simulink model "NEM_DVPP_OPEN"  (R2024a)
settings: Solver=ode23tb  StartTime=0.0  StopTime=60  RelTol=1e-3
libraries: simulink x1
settings Model: Creator=aidan  LastModifiedBy=aidan

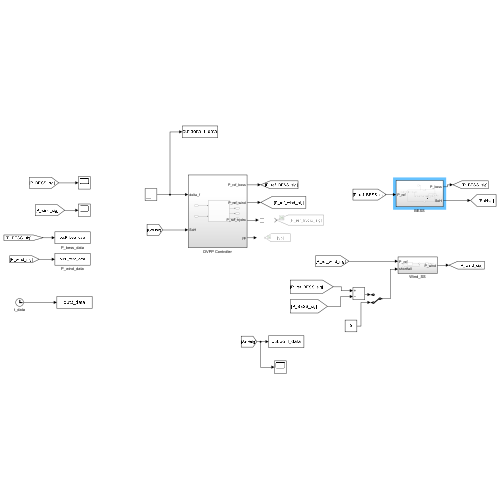
[thumbnail: Simulink's stored preview of the top-level diagram]
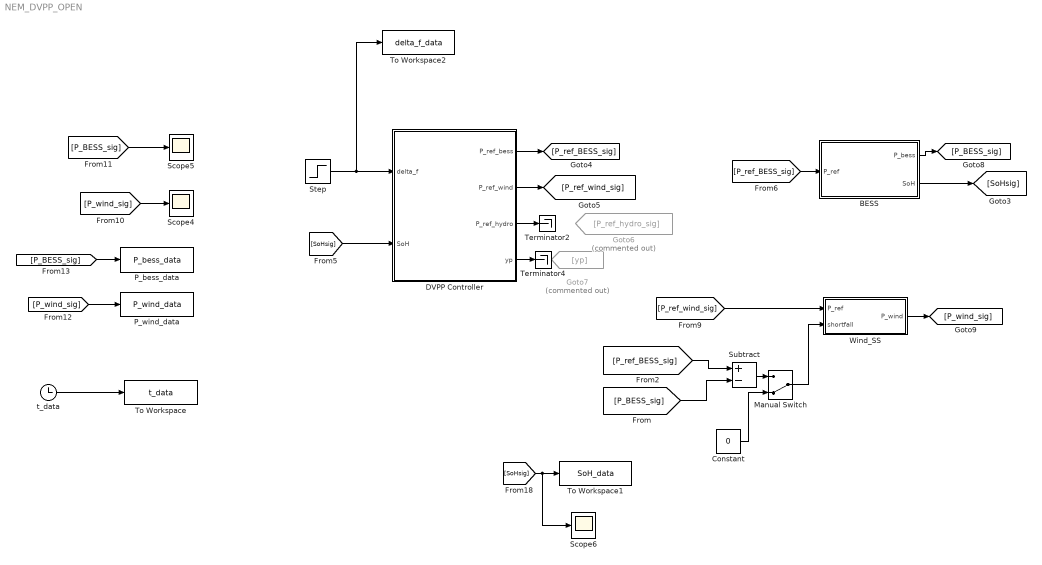
== system NEM_DVPP_OPEN ==
  BESS : Subsystem
  Constant : Constant  Value=0
  DVPP Controller : Subsystem
  Goto6 : Goto  Commented=on  GotoTag=P_ref_hydro_sig
  Goto7 : Goto  Commented=on  GotoTag=yp
  Manual Switch : ManualSwitch  CurrentSetting=0
  P_bess_data : ToWorkspace  VariableName=P_bess_data  SampleTime=-1
  P_wind_data : ToWorkspace  VariableName=P_wind_data  SampleTime=-1
  Scope4 : Scope
  Scope5 : Scope
  Scope6 : Scope
  Step : Step  After=0.75  SampleTime=0
  Subtract : Sum  Inputs=+-
  Terminator2 : Terminator
  Terminator4 : Terminator
  To Workspace : ToWorkspace  VariableName=t_data  SampleTime=-1
  To Workspace1 : ToWorkspace  VariableName=SoH_data  SaveFormat=Timeseries  SampleTime=-1
  To Workspace2 : ToWorkspace  VariableName=delta_f_data  SaveFormat=Timeseries  SampleTime=-1
  Wind_SS : Subsystem
  t_data : Clock
  wires:
  [SoHsig] -> DVPP Controller/2(SoH)
  BESS/2(SoH) -> [SoHsig]
  DVPP Controller/1(P_ref_bess) -> [P_ref_BESS_sig]
  [P_ref_BESS_sig] -> BESS/1(P_ref)
  DVPP Controller/4(yp) -> Terminator4/1
  BESS/1(P_bess) -> [P_BESS_sig]
  DVPP Controller/2(P_ref_wind) -> [P_ref_wind_sig]
  Wind_SS/1(P_wind) -> [P_wind_sig]
  [P_wind_sig] -> Scope4/1
  [P_BESS_sig] -> Scope5/1
  [P_BESS_sig] -> P_bess_data/1
  [P_wind_sig] -> P_wind_data/1
  t_data/1 -> To Workspace/1
  DVPP Controller/3(P_ref_hydro) -> Terminator2/1
  Step/1 -> To Workspace2/1, DVPP Controller/1(delta_f)
  [SoHsig] -> Scope6/1, To Workspace1/1
  [P_ref_BESS_sig] -> Subtract/1
  [P_BESS_sig] -> Subtract/2
  [P_ref_wind_sig] -> Wind_SS/1(P_ref)
  Subtract/1 -> Manual Switch/1
  Constant/1 -> Manual Switch/2
  Manual Switch/1 -> Wind_SS/2(shortfall)

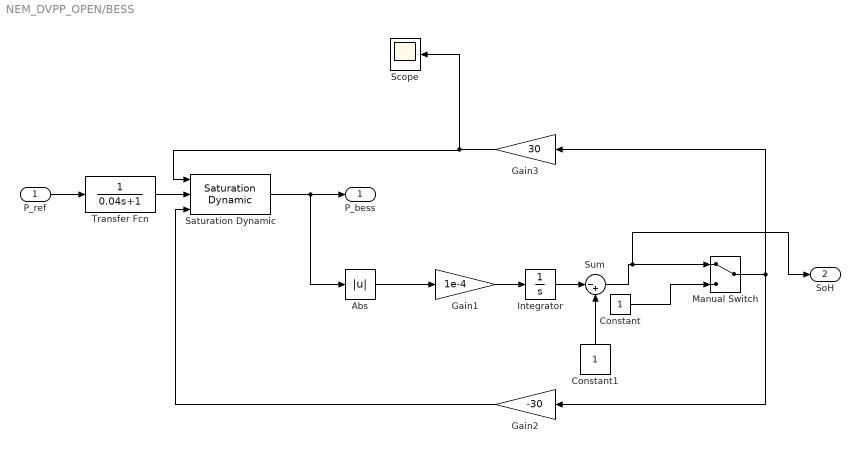
== system NEM_DVPP_OPEN/BESS ==
  P_ref : Inport
  Abs : Abs  SaturateOnIntegerOverflow=off
  Constant : Constant
  Constant1 : Constant
  Gain1 : Gain  Gain=1e-4
  Gain2 : Gain  Gain=-30
  Gain3 : Gain  Gain=30
  Integrator : Integrator
  Manual Switch : ManualSwitch
  Saturation Dynamic : simulink/Discontinuities/Saturation Dynamic  OutMin=[]  OutMax=[]  OutDataTypeStr=Inherit: Same as second input  OutDataType=fixdt(1, 16)  OutScaling=2^-10  DoSatur=off
  Scope : Scope
  Sum : Sum  Inputs=|-+
  Transfer Fcn : TransferFcn  Denominator=[0.04 1]
  P_bess : Outport
  SoH : Outport  Port=2
  wires:
  P_ref/1 -> Transfer Fcn/1
  Saturation Dynamic/1 -> Abs/1, P_bess/1
  Abs/1 -> Gain1/1
  Gain1/1 -> Integrator/1
  Transfer Fcn/1 -> Saturation Dynamic/2
  Constant1/1 -> Sum/2
  Integrator/1 -> Sum/1
  Gain3/1 -> Scope/1, Saturation Dynamic/1
  Sum/1 -> SoH/1, Manual Switch/1
  Constant/1 -> Manual Switch/2
  Manual Switch/1 -> Gain3/1, Gain2/1
  Gain2/1 -> Saturation Dynamic/3

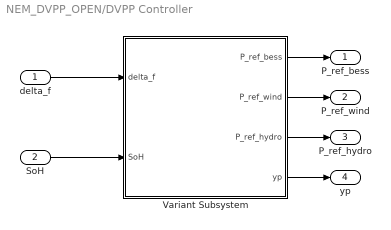
== system NEM_DVPP_OPEN/DVPP Controller ==
  delta_f : Inport
  SoH : Inport  Port=2
  Variant Subsystem : Subsystem  Variant=on
  P_ref_bess : Outport
  P_ref_wind : Outport  Port=2
  P_ref_hydro : Outport  Port=3
  yp : Outport  Port=4
  wires:
  delta_f/1 -> Variant Subsystem/1(delta_f)
  SoH/1 -> Variant Subsystem/2(SoH)
  Variant Subsystem/1(P_ref_bess) -> P_ref_bess/1
  Variant Subsystem/2(P_ref_wind) -> P_ref_wind/1
  Variant Subsystem/3(P_ref_hydro) -> P_ref_hydro/1
  Variant Subsystem/4(yp) -> yp/1

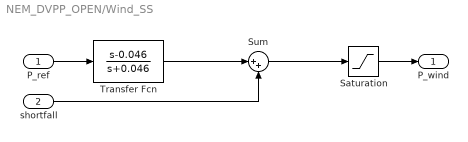
== system NEM_DVPP_OPEN/Wind_SS ==
  P_ref : Inport
  shortfall : Inport  Port=2
  Saturation : Saturate  UpperLimit=20  LowerLimit=-20
  Sum : Sum  Inputs=|++
  Transfer Fcn : TransferFcn  Numerator=[1 -0.046]  Denominator=[1 0.046]
  P_wind : Outport
  wires:
  P_ref/1 -> Transfer Fcn/1
  Saturation/1 -> P_wind/1
  Transfer Fcn/1 -> Sum/1
  Sum/1 -> Saturation/1
  shortfall/1 -> Sum/2

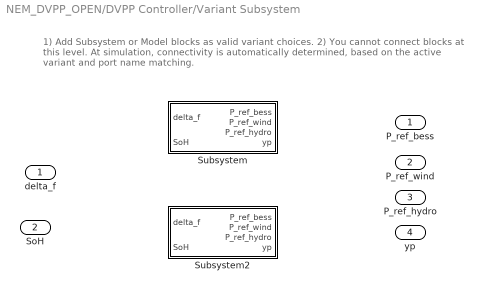
== system NEM_DVPP_OPEN/DVPP Controller/Variant Subsystem ==
  note: 1) Add Subsystem or Model blocks as valid variant choices.
      | 2) You cannot connect blocks at this level. At simulation, connectivity is automatically
      | determined, based on the active variant and port name matching.
  delta_f : Inport
  SoH : Inport  Port=2
  Subsystem : Subsystem  VariantControl=DVPP_MODE == 1
  Subsystem2 : Subsystem  VariantControl=DVPP_MODE == 2
  P_ref_bess : Outport
  P_ref_wind : Outport  Port=2
  P_ref_hydro : Outport  Port=3
  yp : Outport  Port=4

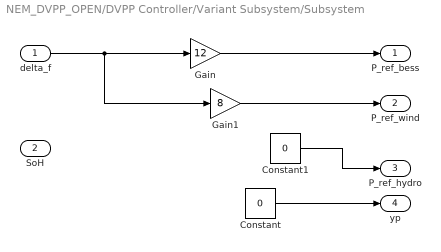
== system NEM_DVPP_OPEN/DVPP Controller/Variant Subsystem/Subsystem ==
  delta_f : Inport
  SoH : Inport  Port=2
  Constant : Constant  Value=0
  Constant1 : Constant  Value=0
  Gain : Gain  Gain=12
  Gain1 : Gain  Gain=8
  P_ref_bess : Outport
  P_ref_wind : Outport  Port=2
  P_ref_hydro : Outport  Port=3
  yp : Outport  Port=4
  wires:
  delta_f/1 -> Gain1/1, Gain/1
  Gain/1 -> P_ref_bess/1
  Gain1/1 -> P_ref_wind/1
  Constant1/1 -> P_ref_hydro/1
  Constant/1 -> yp/1

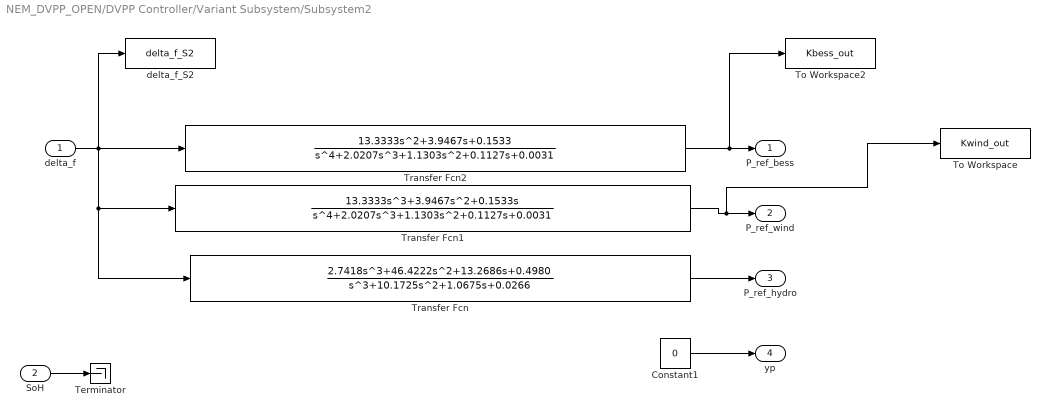
== system NEM_DVPP_OPEN/DVPP Controller/Variant Subsystem/Subsystem2 ==
  delta_f : Inport
  SoH : Inport  Port=2
  Constant1 : Constant  Value=0
  Terminator : Terminator
  To Workspace : ToWorkspace  VariableName=Kwind_out  SaveFormat=Timeseries  SampleTime=-1
  To Workspace2 : ToWorkspace  VariableName=Kbess_out  SaveFormat=Timeseries  SampleTime=-1
  Transfer Fcn : TransferFcn  Numerator=[2.7418, 46.4222, 13.2686, 0.4980]  Denominator=[1, 10.1725, 1.0675, 0.0266]
  Transfer Fcn1 : TransferFcn  Numerator=[13.3333, 3.9467, 0.1533, 0]  Denominator=[1, 2.0207, 1.1303, 0.1127, 0.0031]
  Transfer Fcn2 : TransferFcn  Numerator=[13.3333, 3.9467, 0.1533]  Denominator=[1, 2.0207, 1.1303, 0.1127, 0.0031]
  delta_f_S2 : ToWorkspace  VariableName=delta_f_S2  SaveFormat=Timeseries  SampleTime=-1
  P_ref_bess : Outport
  P_ref_wind : Outport  Port=2
  P_ref_hydro : Outport  Port=3
  yp : Outport  Port=4
  wires:
  delta_f/1 -> delta_f_S2/1, Transfer Fcn2/1, Transfer Fcn/1, Transfer Fcn1/1
  Transfer Fcn2/1 -> To Workspace2/1, P_ref_bess/1
  Transfer Fcn1/1 -> To Workspace/1, P_ref_wind/1
  SoH/1 -> Terminator/1
  Constant1/1 -> yp/1
  Transfer Fcn/1 -> P_ref_hydro/1
